simulink model "DC_Motor_1"  (R2016a)
settings: Solver=VariableStepAuto  StartTime=0.0  StopTime=3.0  RelTol=1e-3
undefined symbols (not defined in the file): b, J, Ke, Kt, L, R
settings Model: Creator=mmdclm  LastModifiedBy=Lara

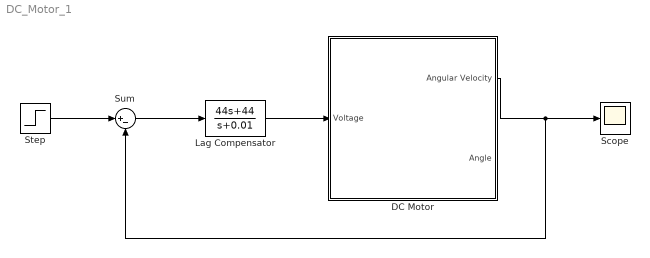
== system DC_Motor_1 ==
  "DC Motor " : Subsystem
  Lag Compensator : TransferFcn  Numerator=[44 44]  Denominator=[1 0.01]
  Scope : Scope
  Step : Step  Time=0  SampleTime=0
  Sum : Sum  Inputs=|+-
  wires:
  "DC Motor "/1(Angular Velocity) -> Sum/2, Scope/1
  Step/1 -> Sum/1
  Lag Compensator/1 -> "DC Motor "/1(Voltage)
  Sum/1 -> Lag Compensator/1

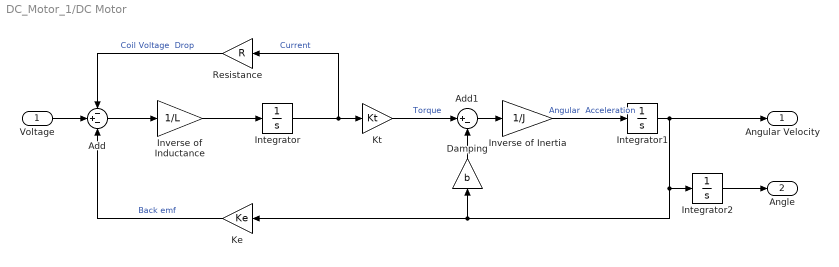
== system DC_Motor_1/DC Motor  ==
  Voltage : Inport
  Add : Sum  Inputs=-+-
  Add1 : Sum  Inputs=|+-
  Damping : Gain  Gain=b
  Integrator : Integrator
  Integrator1 : Integrator
  Integrator2 : Integrator
  Inverse of Inductance : Gain  Gain=1/L
  "Inverse of Inertia " : Gain  Gain=1/J
  "Ke " : Gain  Gain=Ke
  "Kt " : Gain  Gain=Kt
  "Resistance " : Gain  Gain=R
  Angular Velocity : Outport
  Angle : Outport  Port=2
  wires:
  Voltage/1 -> Add/2
  Add/1 -> Inverse of Inductance/1
  "Inverse of Inertia "/1 -> Integrator1/1  "Angular  Acceleration"
  Integrator/1 -> "Kt "/1, "Resistance "/1  "Current"
  "Ke "/1 -> Add/3  "Back emf"
  Inverse of Inductance/1 -> Integrator/1
  Integrator1/1 -> Angular Velocity/1, "Ke "/1, Damping/1, Integrator2/1
  "Resistance "/1 -> Add/1  "Coil Voltage  Drop"
  "Kt "/1 -> Add1/1  "Torque"
  Add1/1 -> "Inverse of Inertia "/1
  Damping/1 -> Add1/2
  Integrator2/1 -> Angle/1
